simulink model "vrmaglev_rtwin"  (Simulink 7.4)
settings: Solver=ode5  SolverMode=SingleTasking  StartTime=0.0  StopTime=Inf  FixedStep=1e-3  MaxStep=0.001  RelTol=1e-3  AbsTol=1e-5
PreLoadFcn:
  | Ts=1e-3;
PostLoadFcn:
  | if ~exist('dsparch4','file') errordlg('Signal Processing Blockset is required to run this demo.', 'Signal Processing Blockset required'); elseif ~exist('rtwinlib','file') errordlg('Real-Time Windows Target is required to run this demo.', 'Real-Time Windows Target required'); end
undefined symbols (not defined in the file or in its folder): Humusoft, MF624
libraries: simulink x3, rtwinlib x2, vrlib x2, dsparch4 x1
Description:
  | Magnetic Levitation Model for Real-Time Windows Target(TM)
  | 
  | In addition to the vrmaglev example, the vrmaglev_rtwin example works directly
  | with the actual CE 152 scale model hardware in real time. We created this model
  | to work with Real Time Workshop, Real-Time Windows Target,
  | and the HUMUSOFT(R) MF 624 multifunction I/O board. However, you can adapt
  | this model for other targets and acquisition boards.
  | 
  | A digital IIR filter, from Signal Processing Toolbox(TM), filters the physical system output.
  | You can bypass the physical system by using the built-in plant model.
  | 
  | Running this model in real time is an example showing the capabilities of Simulink(R)
  | in control systems design and rapid prototyping. When you push the real ball up or down
  | against the coil force, the position of the virtual ball changes in the virtual world.
  | If you remove the ball from the real system, the ball also disappears from the virtual world.
  | The changes to the real system are reflected in real time in its virtual reality representation.
  | 
  | Note that after enabling the remote view in the VR Sink block dialog box, you can visualize
  | the Simulink model even at a remote client computer. This can be useful for distributing
  | the computing power between a real-time Simulink model running on one machine and
  | the rendering of a virtual reality world on another machine.
  | 
  | Note: This demo requires the following software and hardware components:
  | 
  |     * Real Time Workshop
  |     * Real-Time Windows Target(TM)
  |     * Signal Processing Toolbox
  |     * Signal Processing Blockset(TM)
  |     * CE 152 Magnetic Levitation scale model (optional).
  | 
  | More information on the scale model hardware can be found at:
  | http://www.humusoft.com/link/models
settings Model: Creator=Sehnal  LastModifiedBy=Houska  SimulationMode=external  CovMetricSettings=d  ExtModeTrigDuration=5000  ExtModeTrigLevel=0.500000  BufferReuse=off
settings DataIOCC: SaveOutput=off  SaveTime=off  SignalLoggingName=logsOut
settings OptimizationCC: BlockReduction=off  BooleanDataType=off  InlineInvariantSignals=on  OptimizeBlockIOStorage=off  BufferReuse=off  ExpressionFolding=off  LocalBlockOutputs=off  InitFltsAndDblsToZero=on
settings DebuggingCC: CheckExecutionContextPreStartOutputMsg=on  CheckExecutionContextRuntimeOutputMsg=on  SignalResolutionControl=TryResolveAllWithWarning  SolverPrmCheckMsg=none  MultiTaskDSMMsg=warning  MultiTaskCondExecSysMsg=none  StrictBusMsg=None
settings HardwareCC: TargetUnknown=on
settings ModelReferenceCC: UpdateModelReferenceTargets=IfOutOfDate
settings SFSimCC: SimGenerateEmlReport=off
settings RTWCC: SystemTargetFile=rtwin.tlc  TemplateMakefile=rtwin.tmf  RetainRTWFile=on  ProcessScript=rtwin_make_rtw_hook  IncludeERTFirstTime=on
settings RTWinTargetCC: TargetFcnLib=ansi_tfl_tmw.mat  TargetFunctionLibrary=ANSI_C  ModelReferenceCompliant=off  CompOptLevelCompliant=off  MatFileLogging=on  PortableWordSizes=off
settings CustomProperty: DataType=string  Value=on

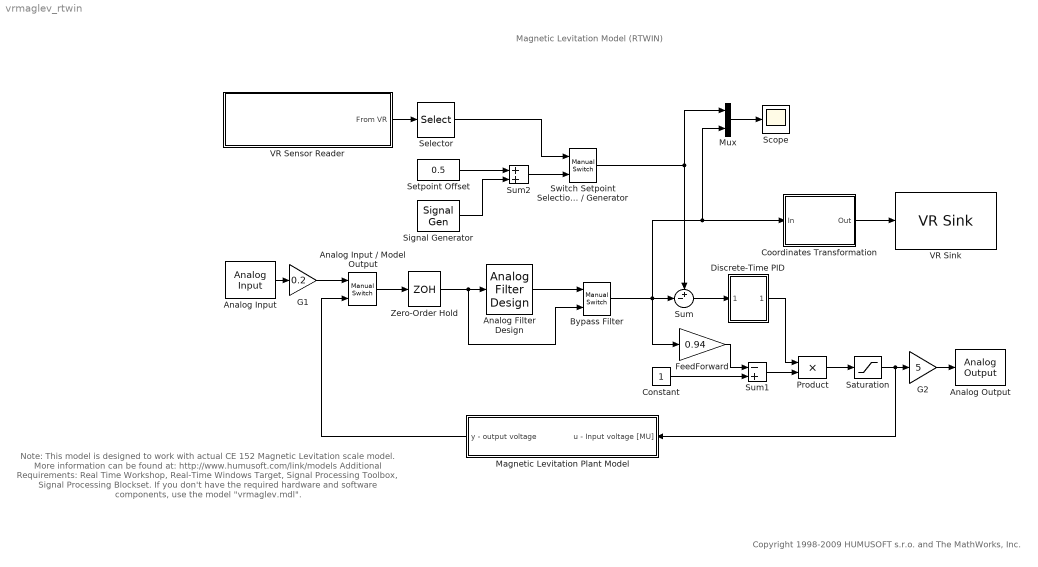
== system vrmaglev_rtwin ==
  note: Magnetic Levitation Model
      | (RTWIN)
  note: Note:
      | This model is designed to work with actual CE 152 Magnetic Levitation scale model. More information can be found at:
      | http://www.humusoft.com/link/models
      | Additional Requirements: Real Time Workshop, Real-Time Windows Target, Signal Processing Toolbox, Signal Processing Blockset.
      | If you don't have the required hardware and software components, use the model "vrmaglev.mdl".
  note: Copyright 1998-2009 HUMUSOFT s.r.o. and The MathWorks, Inc.
  Analog Filter Design : dsparch4/Analog Filter Design  method=Butterworth  filttype=Lowpass  N=2  Wlo=2*pi*100  Whi=80  Rp=2  Rs=40
  Analog Input : rtwinlib/Analog Input  SampleTime=1e-3  DrvName=Humusoft/MF624  DrvAddress=4294967295  DrvOptions=0  Channels=1  RangeMode=1  VoltRange=1  DataType=1
      settings: AttributesFormatString=Humusoft\nMF624 [auto]
  Analog Input / Model Output : simulink/Signal Routing/Manual Switch  SystemSampleTime=-1  sw=1  action=0  varsize=off
  Analog Output : rtwinlib/Analog Output  SampleTime=1e-3  DrvName=Humusoft/MF624  DrvAddress=4294967295  DrvOptions=0  Channels=1  RangeMode=1  VoltRange=1  InitialValue=0  FinalValue=0
      settings: AttributesFormatString=Humusoft\nMF624 [auto]
  Bypass Filter : simulink/Signal Routing/Manual Switch  SystemSampleTime=-1  sw=1  action=0  varsize=off
  Constant : Constant  OutDataType=sfix(16)  OutScaling=2^0
  Coordinates Transformation : Subsystem
  Discrete-Time PID : Subsystem  mask(PID){Kp=1, Ki=10, Kd=0.03, Ts=Ts}
      mask prompts: Ts "Sample time:"
      mask help: Discrete-time PID controller with limited integrator
      mask Display: disp('PID');
  FeedForward : Gain  Gain=0.94  ParameterDataType=sfix(16)  ParameterScaling=2^0  OutDataType=sfix(16)  OutScaling=2^0  SaturateOnIntegerOverflow=on  OutDataTypeStr=Inherit: Same as input  ParamDataTypeStr=Inherit: Same as input
  G1 : Gain  Gain=0.2  ParameterDataType=sfix(16)  ParameterScaling=2^0  OutDataType=sfix(16)  OutScaling=2^0  SaturateOnIntegerOverflow=on  OutDataTypeStr=Inherit: Same as input  ParamDataTypeStr=Inherit: Same as input
  G2 : Gain  Gain=5  ParameterDataType=sfix(16)  ParameterScaling=2^0  OutDataType=sfix(16)  OutScaling=2^0  SaturateOnIntegerOverflow=on  OutDataTypeStr=Inherit: Same as input  ParamDataTypeStr=Inherit: Same as input
  Magnetic Levitation Plant Model : Subsystem
  Mux : Mux  Inputs=2
  Product : Product  OutDataType=sfix(16)  OutScaling=2^0  SaturateOnIntegerOverflow=on  InputSameDT=on  OutDataTypeStr=Inherit: Same as first input
  Saturation : Saturate  UpperLimit=1  LowerLimit=0  ZeroCross=off  OutDataType=sfix(16)  OutScaling=2^0
  Scope : Scope
      settings: TimeRange=5  YMin=-0.0227122  YMax=1.027  DataFormat=Structure  MaxDataPoints=250  SampleInput=on  SampleTime=0.02
  Selector : Selector  InputPortWidth=3  IndexOptions=Index vector (dialog)  Indices=[2]  OutputSizes=1
  Setpoint Offset : Constant  Value=0.5  OutDataType=sfix(16)  OutScaling=2^0
  Signal Generator : SignalGenerator  WaveForm=square  Amplitude=0.2  Frequency=5.0  Units=rad/sec
  Sum : Sum  Inputs=+-|  OutDataType=sfix(16)  OutScaling=2^0  SaturateOnIntegerOverflow=on  InputSameDT=on  OutDataTypeStr=Inherit: Same as first input
  Sum1 : Sum  Inputs=-+  OutDataType=sfix(16)  OutScaling=2^0  SaturateOnIntegerOverflow=on  InputSameDT=on  OutDataTypeStr=Inherit: Same as first input
  Sum2 : Sum  OutDataType=sfix(16)  OutScaling=2^0  SaturateOnIntegerOverflow=on  InputSameDT=on  OutDataTypeStr=Inherit: Same as first input
  Switch Setpoint Selection Method Virtual Reality / Generator : simulink/Signal Routing/Manual Switch  SystemSampleTime=-1  sw=0  action=0  varsize=off
  VR Sensor Reader : Subsystem  mask(VR Sensor Reader){Ts=0.1, vr_world='maglev.wrl', vr_field='Grab_Sensor.translation_changed'}
      mask prompts: Ts "Sample time:"; vr_world "VRML world name:"; vr_field "VRML Node.Field name:"
      mask help: Read value from an exposed VRML field of a VRML scene (usually a VRML sensor output field).
      mask Display: image(imread('vrblockicon.png')); port_label('output', 1, vr_field);
  VR Sink : vrlib/VR Sink  InstantiateOnLoad=on  SampleTime=0.1  ViewEnable=on  RemoteChange=off  RemoteView=off  FieldsWritten=Ball.translation.3.1.double  WorldFileName=maglev.wrl  AutoView=on  VideoDimensions=[]  FigureProperties="{'Position', 'Name', 'Viewpoint', 'CameraBound', 'CameraDirection', 'CameraPosition', 'CameraUpVector', 'ZoomFactor', 'Antialiasing', 'Headlight', 'Lighting', 'NavPanel', 'StatusBar', 'ToolBar', 'Textures', 'Transparency', 'Wireframe', 'NavZones', 'NavMode', 'NavSpeed', 'Record2DCompressMethod', 'Record2DCompressQuality', 'Record2D', 'Record2DFileName', 'Record2DFPS'; [5.0000000000000000e+000  9.2000000000000000e+001  5.7600000000000000e+002  3.8000000000000000e+002], 'VR Magnetic Levitation Model', 'Camera 1', 'on', [0.0000000000000000e+000  4.7981572028401712e-002 -9.9884822107549631e-001], [8.8817841970012523e-016 -7.9831076195052386e-001  1.7287374161691460e-001], [0.0000000000000000e+000  9.9884822107549620e-001  4.7981572028401712e-002], [1.0000000000000000e+000], 'off', 'off', 'on', 'halfbar', 'off', 'on', 'on', 'on', 'off', 'off', 'examine', 'normal', 'auto', [7.5000000000000000e+001], 'off', '%f_anim_%n.avi', [1.5000000000000000e+001]}"
  Zero-Order Hold : ZeroOrderHold  SampleTime=Ts
  wires:
  Constant/1 -> Sum1/2
  Sum1/1 -> Product/2
  FeedForward/1 -> Sum1/1
  Switch Setpoint Selection Method Virtual Reality / Generator/1 -> Sum/1, Mux/1
  Sum/1 -> Discrete-Time PID/1(in_1)
  Discrete-Time PID/1(out_1) -> Product/1
  Mux/1 -> Scope/1
  Product/1 -> Saturation/1
  Analog Input/1 -> G1/1
  Analog Input / Model Output/1 -> Zero-Order Hold/1
  Saturation/1 -> Magnetic Levitation Plant Model/1(u - Input voltage [MU]), G2/1
  Magnetic Levitation Plant Model/1(y - output voltage) -> Analog Input / Model Output/2
  Coordinates Transformation/1(Out) -> VR Sink/1
  G1/1 -> Analog Input / Model Output/1
  G2/1 -> Analog Output/1
  Analog Filter Design/1 -> Bypass Filter/1
  Bypass Filter/1 -> Sum/2, FeedForward/1, Coordinates Transformation/1(In), Mux/2
  Zero-Order Hold/1 -> Analog Filter Design/1, Bypass Filter/2
  Sum2/1 -> Switch Setpoint Selection Method Virtual Reality / Generator/2
  Signal Generator/1 -> Sum2/2
  Setpoint Offset/1 -> Sum2/1
  VR Sensor Reader/1(From VR) -> Selector/1
  Selector/1 -> Switch Setpoint Selection Method Virtual Reality / Generator/1

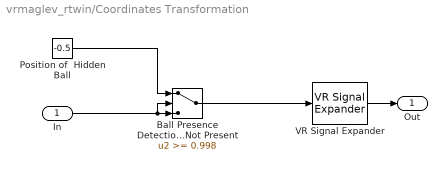
== system vrmaglev_rtwin/Coordinates Transformation ==
  In : Inport  OutDataType=sfix(16)  OutScaling=2^0
  Ball Presence Detection Value > Threshold = Ball Not Present : Switch  Threshold=0.998  OutDataType=sfix(16)  OutScaling=2^0  InputSameDT=on
  Position of  Hidden Ball : Constant  Value=-0.5  OutDataType=sfix(16)  OutScaling=2^0
  VR Signal Expander : vrlib/VR Signal Expander  SystemSampleTime=-1  outwidth=3  outidx=[2]
  Out : Outport  OutDataType=sfix(16)  OutScaling=2^0
  wires:
  Position of  Hidden Ball/1 -> Ball Presence Detection Value > Threshold = Ball Not Present/1
  Ball Presence Detection Value > Threshold = Ball Not Present/1 -> VR Signal Expander/1
  VR Signal Expander/1 -> Out/1
  In/1 -> Ball Presence Detection Value > Threshold = Ball Not Present/3, Ball Presence Detection Value > Threshold = Ball Not Present/2

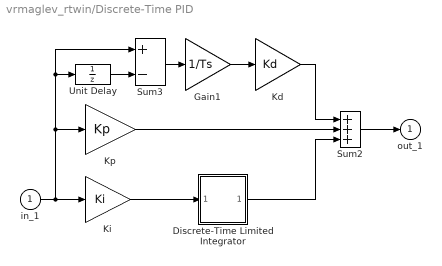
== system vrmaglev_rtwin/Discrete-Time PID ==
  in_1 : Inport  OutDataType=sfix(16)  OutScaling=2^0
  Discrete-Time Limited Integrator : Subsystem  mask(Discrete-Time Limited Integrator.){@1=0, @2=2, @3=0, @4=Ts}
      mask prompts: @1 "Lower bound:"; @2 "Upper bound:"; @3 "Initial condition:"; @4 "Sampling Time:"
      mask help: Discrete-Time Limited Integrator.
      mask init:
      | lower_limit=@1;upper_limit=@2;X0=@3;Ts=@4;
      mask Help: Discrete-Time Limited Integrator. Unmask to see details.
      mask Display: plot(-1,-0.2,3.5,1.2,[0,1,2,2.9],[0,0,1,1],[0,1],[0.5,0.5], [.5,.5], [.8,.6], [.05,.35,.05,.35],[.4,.4,.2,.2], [.45,.65],[.3,.3], [.9,.9],[.2,.4]);
  Gain1 : Gain  Gain=1/Ts  ParameterDataType=sfix(16)  ParameterScaling=2^0  OutDataType=sfix(16)  OutScaling=2^0  SaturateOnIntegerOverflow=on  OutDataTypeStr=Inherit: Same as input  ParamDataTypeStr=Inherit: Same as input
  Kd : Gain  Gain=Kd  ParameterDataType=sfix(16)  ParameterScaling=2^0  OutDataType=sfix(16)  OutScaling=2^0  SaturateOnIntegerOverflow=on  OutDataTypeStr=Inherit: Same as input  ParamDataTypeStr=Inherit: Same as input
  Ki : Gain  Gain=Ki  ParameterDataType=sfix(16)  ParameterScaling=2^0  OutDataType=sfix(16)  OutScaling=2^0  SaturateOnIntegerOverflow=on  OutDataTypeStr=Inherit: Same as input  ParamDataTypeStr=Inherit: Same as input
  Kp : Gain  Gain=Kp  ParameterDataType=sfix(16)  ParameterScaling=2^0  OutDataType=sfix(16)  OutScaling=2^0  SaturateOnIntegerOverflow=on  OutDataTypeStr=Inherit: Same as input  ParamDataTypeStr=Inherit: Same as input
  Sum2 : Sum  Inputs=+++  OutDataType=sfix(16)  OutScaling=2^0  SaturateOnIntegerOverflow=on  InputSameDT=on  OutDataTypeStr=Inherit: Same as first input
  Sum3 : Sum  Inputs=+-  OutDataType=sfix(16)  OutScaling=2^0  SaturateOnIntegerOverflow=on  InputSameDT=on  OutDataTypeStr=Inherit: Same as first input
  Unit Delay : UnitDelay  SampleTime=Ts
  out_1 : Outport  OutDataType=sfix(16)  OutScaling=2^0  InitialOutput=0
  wires:
  Unit Delay/1 -> Sum3/2
  Kd/1 -> Sum2/1
  Kp/1 -> Sum2/2
  Sum2/1 -> out_1/1
  Sum3/1 -> Gain1/1
  Gain1/1 -> Kd/1
  in_1/1 -> Ki/1, Sum3/1, Unit Delay/1, Kp/1
  Ki/1 -> Discrete-Time Limited Integrator/1(in_1)
  Discrete-Time Limited Integrator/1(out_1) -> Sum2/3

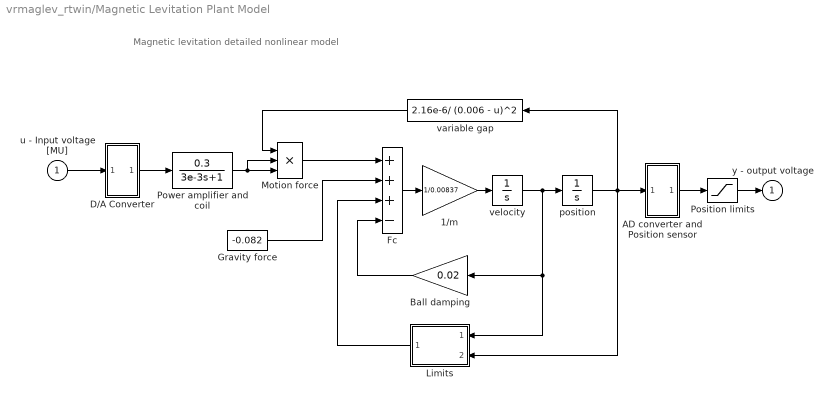
== system vrmaglev_rtwin/Magnetic Levitation Plant Model ==
  note: Magnetic levitation
      | detailed nonlinear model
  u - Input voltage [MU] : Inport  OutDataType=sfix(16)  OutScaling=2^0
  1/m : Gain  Gain=1/0.00837  ParameterDataType=sfix(16)  ParameterScaling=2^0  OutDataType=sfix(16)  OutScaling=2^0  SaturateOnIntegerOverflow=on  OutDataTypeStr=Inherit: Same as input  ParamDataTypeStr=Inherit: Same as input
  AD converter and Position sensor : Subsystem
      mask Display: disp('A/D')
  Ball damping : Gain  Gain=0.02  ParameterDataType=sfix(16)  ParameterScaling=2^0  OutDataType=sfix(16)  OutScaling=2^0  SaturateOnIntegerOverflow=on  OutDataTypeStr=Inherit: Same as input  ParamDataTypeStr=Inherit: Same as input
  D/A Converter : Subsystem
      mask Display: disp('D/A')
  Fc : Sum  Inputs=+++-  OutDataType=sfix(16)  OutScaling=2^0  SaturateOnIntegerOverflow=on  InputSameDT=on  OutDataTypeStr=Inherit: Same as first input
  Gravity force : Constant  Value=-0.082  OutDataType=sfix(16)  OutScaling=2^0
  Limits : Subsystem
      mask Display: disp('LIMIT')
  Motion force : Product  Inputs=3  OutDataType=sfix(16)  OutScaling=2^0  SaturateOnIntegerOverflow=on  InputSameDT=on  OutDataTypeStr=Inherit: Same as first input
  Position limits : Saturate  UpperLimit=0.998  LowerLimit=0  ZeroCross=off  OutDataType=sfix(16)  OutScaling=2^0
  Power amplifier and coil : TransferFcn  Numerator=[0.3]  Denominator=[3e-3 1]
  position : Integrator  LimitOutput=on  UpperSaturationLimit=0.005  LowerSaturationLimit=0  ZeroCross=off
  variable gap : Fcn  Expr=2.16e-6/ (0.006 - u)^2
  velocity : Integrator  UpperSaturationLimit=Inf  LowerSaturationLimit=-Inf  ZeroCross=off
  y - output voltage : Outport  OutDataType=sfix(16)  OutScaling=2^0
  wires:
  velocity/1 -> Ball damping/1, Limits/1(velocity), position/1
  Ball damping/1 -> Fc/4
  variable gap/1 -> Motion force/1
  1/m/1 -> velocity/1
  Fc/1 -> 1/m/1
  Motion force/1 -> Fc/1
  Gravity force/1 -> Fc/2
  D/A Converter/1(out_1) -> Power amplifier and coil/1
  u - Input voltage [MU]/1 -> D/A Converter/1(in_1)
  AD converter and Position sensor/1(out_1) -> Position limits/1
  position/1 -> Limits/2(position), variable gap/1, AD converter and Position sensor/1(in_1)
  Limits/1(force) -> Fc/3
  Power amplifier and coil/1 -> Motion force/3, Motion force/2
  Position limits/1 -> y - output voltage/1

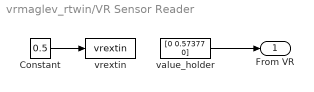
== system vrmaglev_rtwin/VR Sensor Reader ==
  Constant : Constant  Value=0.5  OutDataType=sfix(16)  OutScaling=2^0
  value_holder : Constant  Value="[0     0.57377           0]"  OutDataType=sfix(16)  OutScaling=2^0
  vrextin : S-Function  FunctionName=vrextin  Parameters=Ts, 'maglev.wrl', 'Grab_Sensor.translation_changed'  EnableBusSupport=off
  From VR : Outport  OutDataType=sfix(16)  OutScaling=2^0
  wires:
  value_holder/1 -> From VR/1
  Constant/1 -> vrextin/1

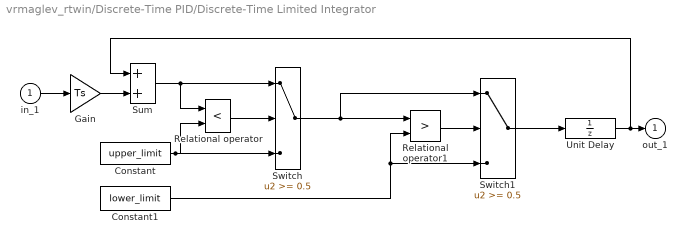
== system vrmaglev_rtwin/Discrete-Time PID/Discrete-Time Limited Integrator ==
  in_1 : Inport  OutDataType=sfix(16)  OutScaling=2^0
  Constant : Constant  Value=upper_limit  OutDataType=sfix(16)  OutScaling=2^0
  Constant1 : Constant  Value=lower_limit  OutDataType=sfix(16)  OutScaling=2^0
  Gain : Gain  Gain=Ts  ParameterDataType=sfix(16)  ParameterScaling=2^0  OutDataType=sfix(16)  OutScaling=2^0  SaturateOnIntegerOverflow=on  OutDataTypeStr=Inherit: Same as input  ParamDataTypeStr=Inherit: Same as input
  Relational operator : RelationalOperator  Operator=<  InputSameDT=on
  Relational operator1 : RelationalOperator  Operator=>  InputSameDT=on
  Sum : Sum  OutDataType=sfix(16)  OutScaling=2^0  SaturateOnIntegerOverflow=on  InputSameDT=on  OutDataTypeStr=Inherit: Same as first input
  Switch : Switch  Threshold=0.5  OutDataType=sfix(16)  OutScaling=2^0  InputSameDT=on
  Switch1 : Switch  Threshold=0.5  OutDataType=sfix(16)  OutScaling=2^0  InputSameDT=on
  Unit Delay : UnitDelay  X0=X0  SampleTime=Ts
  out_1 : Outport  OutDataType=sfix(16)  OutScaling=2^0  InitialOutput=0
  wires:
  Unit Delay/1 -> out_1/1, Sum/1
  Switch1/1 -> Unit Delay/1
  Constant1/1 -> Relational operator1/2, Switch1/3
  Relational operator1/1 -> Switch1/2
  Switch/1 -> Relational operator1/1, Switch1/1
  Constant/1 -> Switch/3, Relational operator/2
  Gain/1 -> Sum/2
  Sum/1 -> Switch/1, Relational operator/1
  Relational operator/1 -> Switch/2
  in_1/1 -> Gain/1

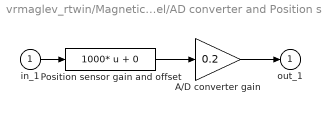
== system vrmaglev_rtwin/Magnetic Levitation Plant Model/AD converter and Position sensor ==
  in_1 : Inport  OutDataType=sfix(16)  OutScaling=2^0
  A/D converter gain : Gain  Gain=0.2  ParameterDataType=sfix(16)  ParameterScaling=2^0  OutDataType=sfix(16)  OutScaling=2^0  SaturateOnIntegerOverflow=on  OutDataTypeStr=Inherit: Same as input  ParamDataTypeStr=Inherit: Same as input
  Position sensor gain and offset : Fcn  Expr=1000* u + 0
  out_1 : Outport  OutDataType=sfix(16)  OutScaling=2^0
  wires:
  in_1/1 -> Position sensor gain and offset/1
  Position sensor gain and offset/1 -> A/D converter gain/1
  A/D converter gain/1 -> out_1/1

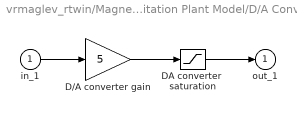
== system vrmaglev_rtwin/Magnetic Levitation Plant Model/D/A Converter ==
  in_1 : Inport  OutDataType=sfix(16)  OutScaling=2^0
  D/A converter gain : Gain  Gain=5  ParameterDataType=sfix(16)  ParameterScaling=2^0  OutDataType=sfix(16)  OutScaling=2^0  SaturateOnIntegerOverflow=on  OutDataTypeStr=Inherit: Same as input  ParamDataTypeStr=Inherit: Same as input
  DA converter  saturation : Saturate  UpperLimit=5  LowerLimit=-5  ZeroCross=off  OutDataType=sfix(16)  OutScaling=2^0
  out_1 : Outport  OutDataType=sfix(16)  OutScaling=2^0
  wires:
  in_1/1 -> D/A converter gain/1
  DA converter  saturation/1 -> out_1/1
  D/A converter gain/1 -> DA converter  saturation/1

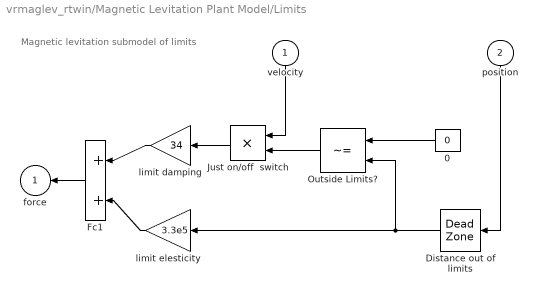
== system vrmaglev_rtwin/Magnetic Levitation Plant Model/Limits ==
  note: Magnetic levitation
      | submodel of limits
  velocity : Inport  OutDataType=sfix(16)  OutScaling=2^0
  position : Inport  Port=2  OutDataType=sfix(16)  OutScaling=2^0
  0 : Constant  Value=0  OutDataType=sfix(16)  OutScaling=2^0
  Distance out of limits : DeadZone  LowerValue=0  UpperValue=0.005  ZeroCross=off  SaturateOnIntegerOverflow=on
  Fc1 : Sum  OutDataType=sfix(16)  OutScaling=2^0  SaturateOnIntegerOverflow=on  InputSameDT=on  OutDataTypeStr=Inherit: Same as first input
  "Just on/off  switch " : Product  OutDataType=sfix(16)  OutScaling=2^0  SaturateOnIntegerOverflow=on  InputSameDT=on  OutDataTypeStr=Inherit: Same as first input
  Outside Limits? : RelationalOperator  Operator=~=  InputSameDT=on
  limit damping : Gain  Gain=34  ParameterDataType=sfix(16)  ParameterScaling=2^0  OutDataType=sfix(16)  OutScaling=2^0  SaturateOnIntegerOverflow=on  OutDataTypeStr=Inherit: Same as input  ParamDataTypeStr=Inherit: Same as input
  limit elesticity : Gain  Gain=3.3e5  ParameterDataType=sfix(16)  ParameterScaling=2^0  OutDataType=sfix(16)  OutScaling=2^0  SaturateOnIntegerOverflow=on  OutDataTypeStr=Inherit: Same as input  ParamDataTypeStr=Inherit: Same as input
  force : Outport  OutDataType=sfix(16)  OutScaling=2^0
  wires:
  Distance out of limits/1 -> Outside Limits?/2, limit elesticity/1
  limit damping/1 -> Fc1/1
  limit elesticity/1 -> Fc1/2
  Outside Limits?/1 -> "Just on/off  switch "/2
  0/1 -> Outside Limits?/1
  "Just on/off  switch "/1 -> limit damping/1
  velocity/1 -> "Just on/off  switch "/1
  Fc1/1 -> force/1
  position/1 -> Distance out of limits/1
